simulink model "model2"  (R2019b)
settings: Solver=VariableStepAuto  StartTime=0.0  StopTime=10.0  RelTol=1e-3
values from neighbouring files (symbols this model uses):
  a = X(1)    [optymalizacja.m]    (also in zad2.m = parametry(1))
  b = X(2)    [optymalizacja.m]    (also in zad2.m = parametry(2))
undefined symbols (not defined in the file or in its folder): licz, licz_in, mian, mian_in
settings Model: Creator=Szymon  LastModifiedBy=Szymon

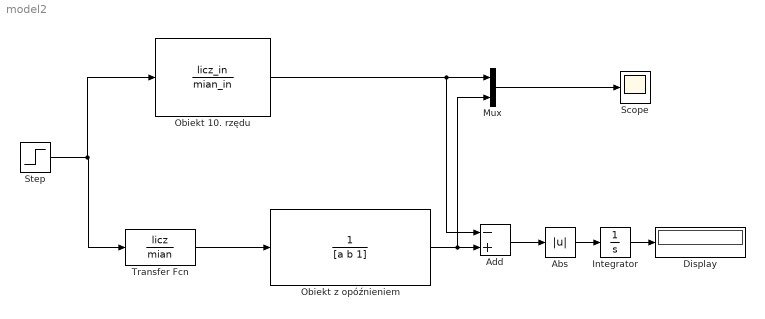
== system model2 ==
  Abs : Abs
  Add : Sum  Inputs=-+
  Display : Display
  Integrator : Integrator
  Mux : Mux  Inputs=2
  Obiekt 10. rzędu : TransferFcn  Numerator=licz_in  Denominator=mian_in
  Obiekt z opóźnieniem : TransferFcn  Denominator=[a b 1]
  Scope : Scope
  Step : Step  Time=0  SampleTime=0
  Transfer Fcn : TransferFcn  Numerator=licz  Denominator=mian
  wires:
  Transfer Fcn/1 -> Obiekt z opóźnieniem/1
  Step/1 -> Obiekt 10. rzędu/1, Transfer Fcn/1
  Mux/1 -> Scope/1
  Obiekt 10. rzędu/1 -> Add/1, Mux/1
  Obiekt z opóźnieniem/1 -> Mux/2, Add/2
  Add/1 -> Abs/1
  Abs/1 -> Integrator/1
  Integrator/1 -> Display/1
